simulink model "dc_shunt_withAR_sim"  (R2020a)
settings: Solver=VariableStepAuto  StartTime=0.0  StopTime=5  RelTol=1e-3
values from neighbouring files (symbols this model uses):
  Ia = [-40:5:40]    [dc_shunt_withAR.m]
  la = 0.018    [dc_shunt_withAR.m]
  lf = 10    [dc_shunt_withAR.m]
  ra = 0.24    [dc_shunt_withAR.m]
  rf = 111    [dc_shunt_withAR.m]
  rload = 1e6    (= 1000000)    [dc_shunt_withAR.m]
  rrh = 25    [dc_shunt_withAR.m]
  vbrush = 2    [dc_shunt_withAR.m]
  wmo = 2000*(2*pi)/60    (= 209.439510239)    [dc_shunt_withAR.m]
  wmrated = 1750*(2*pi)/60    (= 183.259571459)    [dc_shunt_withAR.m]
settings Model: Creator=N SRIKRISHNA  LastModifiedBy=N SRIKRISHNA
settings DataIOCC: ReturnWorkspaceOutputs=off

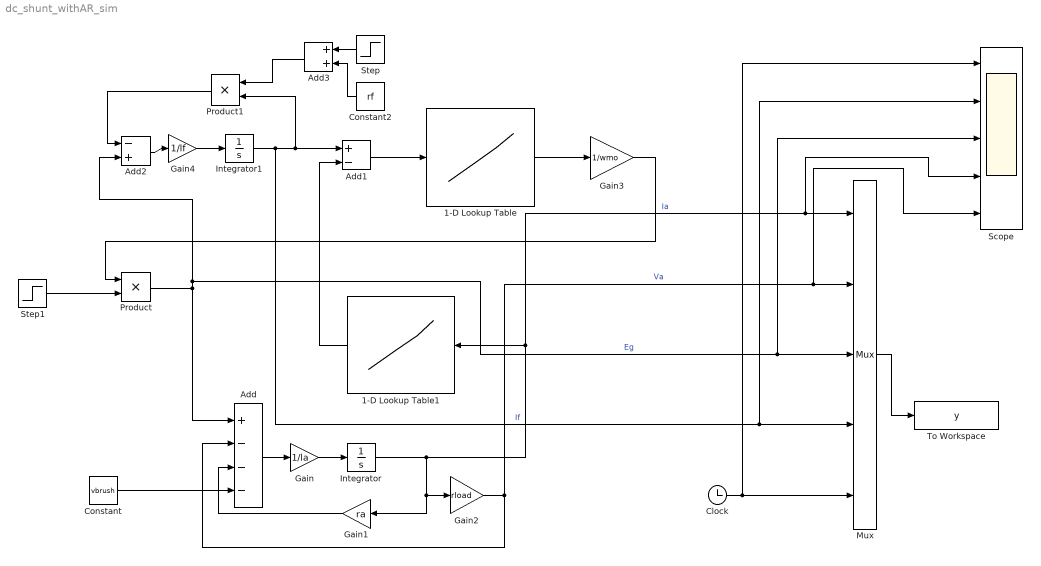
== system dc_shunt_withAR_sim ==
  1-D Lookup Table : Lookup_n-D  NumberOfTableDimensions=1  BreakpointsForDimension1=[0 0.05 0.1 0.13 0.18 0.22 0.26 0.32 0.36 0.4 0.47 0.54 0.575 0.61 0.64 0.68 0.71 0.74 0.78 0.82 0.86 0.9 0.93 1.0 1.1 1.2 1.3 1.4 1.5]  Table=[7.5 12 20 24 32 40 48 59 66 74 86 97 102.5 107.5 112 117 121 125 130 135 140 143 146 152 158 164 168 172 175]  InternalRulePriority=Speed  RndMeth=Simplest  InputSameDT=on
  1-D Lookup Table1 : Lookup_n-D  NumberOfTableDimensions=1  BreakpointsForDimension1=Ia  Table=0.04*abs(atan(Ia)) + 0.0001*Ia.^2  InternalRulePriority=Speed  RndMeth=Simplest  InputSameDT=on
  Add : Sum  Inputs=+---
  Add1 : Sum  Inputs=+-
  Add2 : Sum  Inputs=-+
  Add3 : Sum
  Clock : Clock
  Constant : Constant  Value=vbrush
  Constant2 : Constant  Value=rf
  Gain : Gain  Gain=1/la
  Gain1 : Gain  Gain=ra
  Gain2 : Gain  Gain=rload
  Gain3 : Gain  Gain=1/wmo
  Gain4 : Gain  Gain=1/lf
  Integrator : Integrator
  Integrator1 : Integrator
  Mux : Mux  Inputs=5
  Product : Product
  Product1 : Product
  Scope : Scope  NumInputPorts=5
  Step : Step  Time=10  Before=rrh  After=0  SampleTime=0
  Step1 : Step  Time=0  After=wmrated  SampleTime=0
  To Workspace : ToWorkspace  VariableName=y  SampleTime=-1
  wires:
  Constant/1 -> Add/4
  Add/1 -> Gain/1
  Gain/1 -> Integrator/1
  Integrator/1 -> Gain2/1, Gain1/1, Scope/4, Mux/1, 1-D Lookup Table1/1  "Ia"
  Gain1/1 -> Add/3
  Gain2/1 -> Add/2, Scope/5, Mux/2  "Va"
  1-D Lookup Table1/1 -> Add1/2
  Add1/1 -> 1-D Lookup Table/1
  1-D Lookup Table/1 -> Gain3/1
  Step1/1 -> Product/2
  Gain3/1 -> Product/1
  Product/1 -> Scope/3, Mux/3, Add2/2, Add/1  "Eg"
  Add2/1 -> Gain4/1
  Gain4/1 -> Integrator1/1
  Integrator1/1 -> Product1/2, Add1/1, Scope/2, Mux/4  "If"
  Product1/1 -> Add2/1
  Clock/1 -> Scope/1, Mux/5
  Mux/1 -> To Workspace/1
  Step/1 -> Add3/1
  Constant2/1 -> Add3/2
  Add3/1 -> Product1/1
